simulink library "csc_hio_hardware_io_lib"  (R2014b)
settings: Solver=ode45  StartTime=0.0  StopTime=10.0  RelTol=1e-3
values from neighbouring files (symbols this model uses):
  fsw_dt = 0.1    [csci_fsw_init.m]
libraries: util_info_lib x1, util_common_lib x1
settings Model: Creator=mstewart  LastModifiedBy=mstewart

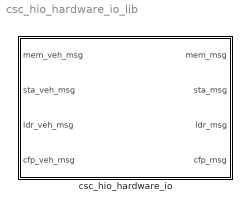
== system csc_hio_hardware_io_lib ==
  csc_hio_hardware_io : Subsystem  TreatAsAtomicUnit=on  SystemSampleTime=fsw_dt

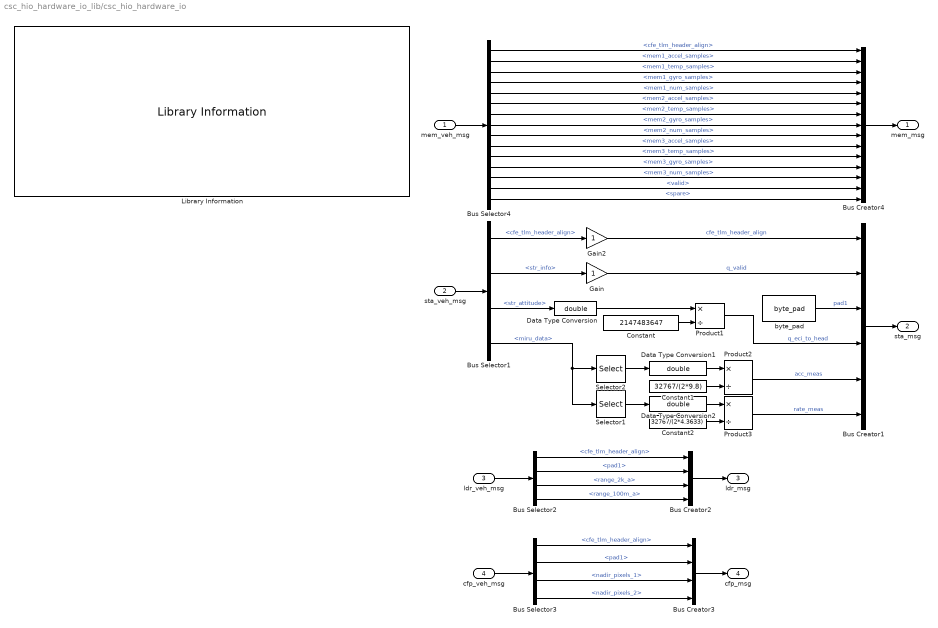
== system csc_hio_hardware_io_lib/csc_hio_hardware_io ==
  mem_veh_msg : Inport
  sta_veh_msg : Inport  Port=2
  ldr_veh_msg : Inport  Port=3  OutDataTypeStr=Bus: ldr_veh_msg
  cfp_veh_msg : Inport  Port=4  OutDataTypeStr=Bus: cfp_veh_msg
  Bus Creator1 : BusCreator  Inputs=6  OutDataTypeStr=Bus: sta_msg  NonVirtualBus=on
  Bus Creator2 : BusCreator  OutDataTypeStr=Bus: ldr_msg  NonVirtualBus=on
  Bus Creator3 : BusCreator  OutDataTypeStr=Bus: cfp_msg  NonVirtualBus=on
  Bus Creator4 : BusCreator  Inputs=15  OutDataTypeStr=Bus: mem_msg  NonVirtualBus=on
  Bus Selector1 : BusSelector  OutputSignals=fused_attitude.cfe_tlm_header_align,fused_attitude.str_info,fused_attitude.str_attitude,miru_data.miru_data
  Bus Selector2 : BusSelector  OutputSignals=cfe_tlm_header_align,pad1,range_2k_a,range_100m_a
  Bus Selector3 : BusSelector  OutputSignals=cfe_tlm_header_align,pad1,nadir_pixels_1,nadir_pixels_2
  Bus Selector4 : BusSelector  OutputSignals=cfe_tlm_header_align,mem1_accel_samples,mem1_temp_samples,mem1_gyro_samples,mem1_num_samples,mem2_accel_samples,mem2_temp_samples,mem2_gyro_samples,mem2_num_samples,mem3_accel_samples,mem3_temp_samples,mem3_gyro_samples,mem3_num_samples,valid,spare
  Constant : Constant  Value=2147483647  OutDataTypeStr=double
  Constant1 : Constant  Value=32767/(2*9.8)  OutDataTypeStr=double
  Constant2 : Constant  Value=32767/(2*4.3633)  OutDataTypeStr=double
  Data Type Conversion : DataTypeConversion  OutDataTypeStr=double
  Data Type Conversion1 : DataTypeConversion  OutDataTypeStr=double
  Data Type Conversion2 : DataTypeConversion  OutDataTypeStr=double
  Gain : Gain  OutDataTypeStr=uint8
  Gain2 : Gain  OutDataTypeStr=uint8
  Library Information : util_info_lib/Library Information  owner='NONE'
  Product1 : Product  Inputs=*/  RndMeth=Zero
  Product2 : Product  Inputs=*/  RndMeth=Zero
  Product3 : Product  Inputs=*/  RndMeth=Zero
  Selector1 : Selector  NumberOfDimensions=2  InputPortWidth=11  IndexOptions=Select all,Index vector (dialog)  Indices=1,[9 10 11]  OutputSizes=1,1
  Selector2 : Selector  NumberOfDimensions=2  InputPortWidth=11  IndexOptions=Select all,Index vector (dialog)  Indices=1,[1:8]  OutputSizes=1,1
  byte_pad : util_common_lib/byte_pad  n_bytes=3
  mem_msg : Outport  OutDataTypeStr=Bus: mem_msg
  sta_msg : Outport  Port=2  OutDataTypeStr=Bus: sta_msg
  ldr_msg : Outport  Port=3  OutDataTypeStr=Bus: ldr_msg
  cfp_msg : Outport  Port=4  OutDataTypeStr=Bus: cfp_msg
  wires:
  Bus Selector4/12 -> Bus Creator4/12  "<mem3_gyro_samples>"
  Bus Selector4/13 -> Bus Creator4/13  "<mem3_num_samples>"
  Bus Selector4/15 -> Bus Creator4/15  "<spare>"
  Bus Selector4/11 -> Bus Creator4/11  "<mem3_temp_samples>"
  Bus Selector4/14 -> Bus Creator4/14  "<valid>"
  Bus Selector4/10 -> Bus Creator4/10  "<mem3_accel_samples>"
  Bus Selector4/9 -> Bus Creator4/9  "<mem2_num_samples>"
  Bus Selector4/8 -> Bus Creator4/8  "<mem2_gyro_samples>"
  Bus Selector4/7 -> Bus Creator4/7  "<mem2_temp_samples>"
  Bus Selector4/6 -> Bus Creator4/6  "<mem2_accel_samples>"
  Bus Selector4/5 -> Bus Creator4/5  "<mem1_num_samples>"
  Bus Selector4/4 -> Bus Creator4/4  "<mem1_gyro_samples>"
  Bus Selector4/3 -> Bus Creator4/3  "<mem1_temp_samples>"
  Bus Selector4/2 -> Bus Creator4/2  "<mem1_accel_samples>"
  Bus Selector4/1 -> Bus Creator4/1  "<cfe_tlm_header_align>"
  Bus Creator4/1 -> mem_msg/1
  mem_veh_msg/1 -> Bus Selector4/1
  Selector1/1 -> Data Type Conversion2/1
  Data Type Conversion2/1 -> Product3/1
  Constant2/1 -> Product3/2
  Selector2/1 -> Data Type Conversion1/1
  Data Type Conversion1/1 -> Product2/1
  Constant1/1 -> Product2/2
  Data Type Conversion/1 -> Product1/1
  Constant/1 -> Product1/2
  Gain2/1 -> Bus Creator1/1  "cfe_tlm_header_align"
  Product2/1 -> Bus Creator1/5  "acc_meas"
  Bus Selector1/4 -> Selector2/1, Selector1/1  "<miru_data>"
  Product1/1 -> Bus Creator1/4  "q_eci_to_head"
  Gain/1 -> Bus Creator1/2  "q_valid"
  Bus Selector3/1 -> Bus Creator3/1  "<cfe_tlm_header_align>"
  Bus Selector2/1 -> Bus Creator2/1  "<cfe_tlm_header_align>"
  Bus Selector1/1 -> Gain2/1  "<cfe_tlm_header_align>"
  byte_pad/1 -> Bus Creator1/3  "pad1"
  Bus Selector3/4 -> Bus Creator3/4  "<nadir_pixels_2>"
  Bus Selector3/3 -> Bus Creator3/3  "<nadir_pixels_1>"
  Bus Selector3/2 -> Bus Creator3/2  "<pad1>"
  Bus Selector2/4 -> Bus Creator2/4  "<range_100m_a>"
  Bus Selector2/3 -> Bus Creator2/3  "<range_2k_a>"
  Bus Selector2/2 -> Bus Creator2/2  "<pad1>"
  Product3/1 -> Bus Creator1/6  "rate_meas"
  Bus Selector1/3 -> Data Type Conversion/1  "<str_attitude>"
  Bus Selector1/2 -> Gain/1  "<str_info>"
  Bus Creator1/1 -> sta_msg/1
  Bus Creator2/1 -> ldr_msg/1
  Bus Creator3/1 -> cfp_msg/1
  cfp_veh_msg/1 -> Bus Selector3/1
  ldr_veh_msg/1 -> Bus Selector2/1
  sta_veh_msg/1 -> Bus Selector1/1
